simulink model "P_CGMRES_fast"  (R2023a)
settings: Solver=FixedStepAuto  StartTime=0.0  StopTime=22.16  RelTol=1e-3
values from neighbouring files (symbols this model uses):
  lujing = 8    [main.m]
libraries: Solver_SF x1
(part 19 of 21)

== matlab function P_CGMRES_fast/快速有约束罚函数求解同样迭代次数/基于增广拉格朗日1 ==
  settings: updateMethod=DISCRETE
  data: deltaf output size=[10,1]; wref input; vx input; gain2 input
function deltaf = yueshu(wref,vx,gain2)
deltaf=zeros(10,1);
dc=1.55;
for i=1:length(deltaf)
    deltaf(i)=atan(wref.*dc./vx)*gain2;
    % deltaf(i)=wref/5;
end
end

== matlab function P_CGMRES_fast/快速有约束罚函数求解同样迭代次数/基于增广拉格朗日2 ==
  settings: updateMethod=DISCRETE
  data: caltime input; F_final output size=[1,1]; deltaf2 input; vx input; ax input; x_ref input; y_ref input; theta_ref input; omega_ref input; x input; y input; theta input; vx1 input; vy input; omega input; deltaf_lastout input; gain1 output; gain2 output; F_first output; caltime2 output
function [F_final,gain1,gain2,F_first,caltime2] = yueshu(caltime,deltaf2,vx,ax,x_ref,y_ref,theta_ref,omega_ref,x,y,theta,vx1,vy,omega,deltaf_lastout)
tic
%% 初始速度42km/h，如果跟踪效果的提升不明显，调整上下界，二者越接近1效果越好
%% 如果改动了初始的优化变量，需要修改ini_c = ones(SwarmSize,1)*[0.8,0.95];
%% 如果想要更改优化变量去改cc_v和cc_ome
%% 终端约束设置为0，不要改，改的太大会导致控制量飞掉
%%  如果寻优结果总是在边界处，调大除的640000，fSwarm(j,:)=abs(sum(F(:)))/640000;
deltaf=zeros(10,1);
dc=1.55;
Kp=0;
Ka=4000;
omega_min=-0.095;
gain=0;
deltaf=deltaf2+deltaf;
% for i=1:length(deltaf)
%     deltaf(i)=atan(wref.*dc./vx);
%     % deltaf(i)=wref/5;
% end
%% 参数设置
w = 0.6;      % 惯性因子 ---可设置为变化的
cc1 = 2;       % 加速常数
cc2 = 2;       % 加速常数

Dim = 2;            % 维数
SwarmSize = 5;    % 粒子群规模

MaxIter = 50;      % 最大迭代次数  
MinFit = 10000000;       % 最小适应值 

Vmax = 1;
Vmin = -1;
%% 上下界约接近1效果越好
Lb = ([0.9 0]);
Ub = ([1.1 6.5]);


%% 粒子群初始化
    Range = ones(SwarmSize,1)*(Ub-Lb);
    ini_c = ones(SwarmSize,1)*[1,1];%%%%%% 初值
    % Swarm = ini_c.*Range + zeros(SwarmSize,1)*Lb; 
    Swarm = ini_c; 
    % Swarm = rand(SwarmSize,Dim).*Range + ones(SwarmSize,1)*Lb;      % 初始化粒子群
    VStep = rand(SwarmSize,Dim)*(Vmax-Vmin) + Vmin;                 % 初始化速度
    fSwarm = zeros(SwarmSize,1);
for i=1:SwarmSize
% feval()函数执行指定的函数。
% 也就是说，将想要执行的函数以及相应的参数一起作为feval()的参数，
% feval()的输出等于想要执行的函数的输出
   cc_v=ax*Swarm(i,1);
   ccc_ome=deltaf*Swarm(i,2);
   [F]=calF(x_ref,y_ref,theta_ref,omega_ref,x,y,theta,vx,vy,omega,cc_v,ccc_ome,gain,deltaf_lastout,Kp,omega_min,Ka);
   fSwarm(i,:)=abs(sum(F(:)));                        % 粒子群的适应值 
end
F_first=abs(sum(F(:)));
%% 个体极值和群体极值
[bestf bestindex]=min(fSwarm);
zbest=Swarm(bestindex,:);   % 全局最佳
gbest=Swarm;                % 个体最佳
fgbest=fSwarm;              % 个体最佳适应值
fzbest=bestf;               % 全局最佳适应值

%% 迭代寻优
iter = 0;
y_fitness = zeros(1,MaxIter);   % 预先产生4个空矩阵
c1 = zeros(1,MaxIter); %% MaxIter 最大迭代次数        
c2 = zeros(1,MaxIter);
% c1_R = zeros(1,MaxIter); 
% c2_R = zeros(1,MaxIter);

while( (iter < MaxIter) && (fzbest > MinFit) )
    for j=1:SwarmSize
        % 速度更新
        VStep(j,:) = w*VStep(j,:) + cc1*rand*(gbest(j,:) - Swarm(j,:)) + cc2*rand*(zbest - Swarm(j,:));
        if VStep(j,:)>Vmax, VStep(j,:)=Vmax; end
        if VStep(j,:)<Vmin, VStep(j,:)=Vmin; end
        % 位置更新
        Swarm(j,:)=Swarm(j,:)+VStep(j,:);
        for k=1:Dim
            if Swarm(j,k)>Ub(k), Swarm(j,k)=Ub(k); end
            if Swarm(j,k)<Lb(k), Swarm(j,k)=Lb(k); end
        end
        % 适应值
        cc_v=ax*Swarm(i,1);
        ccc_ome=deltaf*Swarm(i,2);
        [F]=calF(x_ref,y_ref,theta_ref,omega_ref,x,y,theta,vx,vy,omega,cc_v,ccc_ome,gain,deltaf_lastout,Kp,omega_min,Ka);
        fSwarm(j,:)=abs(sum(F(:)));
        % 个体最优更新     
        if fSwarm(j) < fgbest(j)
            gbest(j,:) = Swarm(j,:);
            fgbest(j) = fSwarm(j);
        end
        % 群体最优更新
        if fSwarm(j) < fzbest
            zbest = Swarm(j,:);
            fzbest = fSwarm(j);
        end
    end 
    iter = iter+1;                      % 迭代次数更新
    y_fitness(1,iter) = fzbest;         % 为绘图做准备
    c1(1,iter) = zbest(1);
    c2(1,iter) = zbest(2);
end
F_final=fzbest;
caltime2=toc+caltime;
gain1=zbest(1);
gain2=zbest(2);
end

function [F]= calF(x_ref,y_ref,theta_ref,omega_ref,x,y,theta,vx,vy,omega,ax_real,deltaf_real,gain,deltaf_lastout,Kp,omega_min,Ka)

N=10;
V_tar=18;

F=zeros(2*N,1);
F_temp=zeros(2*N,1);

% cc=deltaf_real(1);
% deltaf_real=deltaf_real;
% deltaf_real(1)=cc/5;

x_real=zeros(N,1);
y_real=zeros(N,1);
theta_real=zeros(N,1);
alphaf=zeros(N,1);
alphar=zeros(N,1);
vx_real=zeros(N,1);
vy_real=zeros(N,1);
omega_real=zeros(N,1);





x_real(1)=x;
y_real(1)=y;
theta_real(1)=theta;
vx_real(1)=vx;
vy_real(1)=vy;
omega_real(1)=omega;



dot_x=[];

H_x=zeros(N,1);
H_y=zeros(N,1);
H_theta=zeros(N,1);
H_vx=zeros(N,1);
H_vy=zeros(N,1);
H_omega=zeros(N,1);

H_ax=zeros(N,1);
H_ax_temp=zeros(N,1);
H_deltaf=zeros(N,1);
H_deltaf_temp=zeros(N,1);
P1=zeros(N,1);
P2=zeros(N,1);
P3=zeros(N,1);
P4=zeros(N,1);
P5=zeros(N,1);
P6=zeros(N,1);

%% 参数初始化
Cx=10;
Cy=1000*3*22*1420;
Cvx=90*2500;
Ctheta=500000*0.8*100;
Comega=6000*5;

Cax=60000;
Cdeltaf=15000*498000;
Cdeltadeltaf=150000000000*5*0;
C_stability=10000000*1500;
Delt_T=0.02*3.5;
cf=-90700;
cr=-109000;
lf=1.05;
lr=1.61;
m=1430;
Iz=2059;
h=0.02*3.5;
As=-50/3.5;
error=0;
                                                                                                                                                                                                                                                                                                                                                                                                                                                                                                                                                                                                                                                                                                                                                                                                                                                                                                                                                                                                                                                                                                                                                                                                                                                                                                                                                                                                                                                                                                                                                                                                                                                                                                                                                                                                                                                   


% if x<80
%     Cx=10;
%     Cy=300;
% 
%     Cv=20000*15.6;
% 
%     Ctheta=1000;
%     Comega=6000*5;
%     Cdeltaw=1500000;
% 
%     Cw=300;
% end
% if x>150
%     Cx=10;
%     Cy=800;
% 
%     Cv=20000*15.6;
% 
%     Ctheta=1000;
%     Comega=6000*5;
%     Cdeltaw=1500000;
% 
%     Cw=300;
% end
for i=1:N-1
    %% 更新状态
    alphaf(i)=(vy_real(i)+lf*omega_real(i))/vx_real(i)-deltaf_real(i);
    alphar(i)=(vy_real(i)-lr*omega_real(i))/vx_real(i);
    x_real(i+1) = x_real(i)+Delt_T*(vx_real(i)*cos(theta_real(i))-vy_real(i)*sin(theta_real(i)));
    y_real(i+1) = y_real(i)+Delt_T*(vx_real(i)*sin(theta_real(i))+vy_real(i)*cos(theta_real(i)));
    omega_real(i+1)=omega_real(i)+Delt_T*(2/Iz*(lf*cf*alphaf(i)-lr*cr*alphar(i)));
    theta_real(i+1) = theta_real(i)+Delt_T*omega_real(i);
    vx_real(i+1)=vx_real(i)+Delt_T*(ax_real(i)+vy_real(i)*omega_real(i));
    vy_real(i+1)=vy_real(i)+Delt_T*(-vx_real(i)*omega_real(i)+2/m*(cf*alphaf(i)+cr*alphar(i)));
end

P1(N)=2*0*(x_real(N)-x_ref(N));
P2(N)=2*0*(y_real(N)-y_ref(N));
P3(N)=2*0*(theta_real(N)-theta_ref(N));
P4(N)=2*50*(omega_real(N)-omega_ref(N)-gain);
P5(N)=2*0*(vx_real(N)-V_tar);
P6(N)=2*0*(vy_real(N));
% P1(N)=0;
% P2(N)=0;
% P3(N)=0;
for i=N:-1:2
    H_x(i)=2*Cx*(x_real(i)-x_ref(i));
    H_y(i)=2*Cy*(y_real(i)-y_ref(i));
    H_theta(i)=2*Ctheta*(theta_real(i)-theta_ref(i))+P1(i)*(-vx_real(i)*sin(theta_real(i))-vy_real(i)*cos(theta_real(i)))...
        +P2(i)*(vx_real(i)*cos(theta_real(i))-vy_real(i)*sin(theta_real(i)));
    H_vx(i)=2*Cvx*(vx_real(i)-V_tar)+P1(i)*(cos(theta_real(i)))...
        +P2(i)*(sin(theta_real(i)))...
        +P4(i)*2/Iz*(lf*cf*-(vy_real(i)+lf*omega_real(i))/(vx_real(i)^2)+lr*cr*(vy_real(i)-lr*omega_real(i))/(vx_real(i)^2))...
        +P6(i)*(-omega_real(i)+2/m*(-cf*(vy_real(i)+lf*omega_real(i))/(vx_real(i)^2)-cr*(vy_real(i)-lr*omega_real(i))/(vx_real(i)^2)));
    H_vy(i)=P1(i)*(-sin(theta_real(i)))...
        +P2(i)*(cos(theta_real(i)))...
        +P4(i)*2/Iz*(lf*cf/(vx_real(i))-lr*cr/(vx_real(i)))...
        +P5(i)*omega_real(i)...
        +P6(i)*(2/m*(1*cf/(vx_real(i))+(1*cr)/(vx_real(i))));
    H_omega(i)=2*Comega*(omega_real(i)-omega_ref(i))+P3(i)...
        +P4(i)*2/Iz*(lf*cf*lf/(vx_real(i))+lr*cr*lr/(vx_real(i)))...
        +P5(i)*vy_real(i)...
        +P6(i)*(vx_real(i)+2/m*(lf*cf/(vx_real(i))-(lr*cr)/(vx_real(i))))...
        -Ka*Kp*exp(-Ka*(omega_min-omega_real(i)))/(1+exp(-Ka*(omega_min-omega_real(i))))^2; 

   
    %% 更新协态变量
    P1(i-1) = P1(i) + H_x(i)*Delt_T;
    P2(i-1) = P2(i) + H_y(i)*Delt_T;
    P3(i-1) = P3(i) + H_theta(i)*Delt_T;
    P5(i-1) = P5(i) + H_vx(i)*Delt_T;
    P6(i-1) = P6(i) + H_vy(i)*Delt_T;
    P4(i-1) = P4(i) + H_omega(i)*Delt_T;
end
for i=1:N
    H_ax(i)=2*Cax*(ax_real(i))+P5(i);
    if i==1
        H_deltaf(i)=P4(i)*(2/Iz*lf*cf*-1)+P6(i)*(2/m*cf*-1)+2*Cdeltaf*deltaf_real(i)-2*Cdeltadeltaf*(deltaf_real(i+1)-deltaf_real(i))+2*C_stability*(deltaf_real(i)-deltaf_lastout);
    elseif i==N
        H_deltaf(i)=P4(i)*(2/Iz*lf*cf*-1)+P6(i)*(2/m*cf*-1)+2*Cdeltaf*deltaf_real(i)+2*Cdeltadeltaf*(deltaf_real(i)-deltaf_real(i-1))+2*C_stability*(deltaf_real(i)-deltaf_lastout);
    else
        H_deltaf(i)=P4(i)*(2/Iz*lf*cf*-1)+P6(i)*(2/m*cf*-1)+2*Cdeltaf*deltaf_real(i)-2*Cdeltadeltaf*(deltaf_real(i+1)-deltaf_real(i))+2*Cdeltadeltaf*(deltaf_real(i)-deltaf_real(i-1))+2*C_stability*(deltaf_real(i)-deltaf_lastout);
    end
    F(2*i-1,1)=H_ax(i);
    F(2*i,1)=H_deltaf(i);
end




% for i=1:N-1
%     %% 更新状态
%     x_real(i+1) = x_real(i)+Delt_T*V_real(i)*cos(theta_real(i));
%     y_real(i+1) = y_real(i)+Delt_T*V_real(i)*sin(theta_real(i));
%     theta_real(i+1) = theta_real(i)+Delt_T*omega_real(i);
% end


end

== matlab function P_CGMRES_fast/快速有约束罚函数求解同样迭代次数/基于增广拉格朗日3 ==
  settings: updateMethod=DISCRETE
  data: ax2 output size=[10,1]; ax input; gain1 input
function ax2 = yueshu(ax,gain1)
ax2=ax*gain1;
end

== matlab function P_CGMRES_fast/Subsystem/MATLAB Function ==
  data: y input; thetaf output; x input
function thetaf = fcn(y,x)

thetaf = atan(y/x);
end

== matlab function P_CGMRES_fast/Subsystem/MATLAB Function1 ==
  data: y input; thetaf output; x input
function thetaf = fcn(y,x)

thetaf = atan(y/x);
end
